simulink model "einMassenSchwingerAngeregt"  (R2017b)
settings: Solver=ode8  StartTime=0.0  StopTime=t_max  FixedStep=stepSize  RelTol=relTol
values from neighbouring files (symbols this model uses):
  c = 10    [Aufgabe2_parameterInit.m]
  d = .5    (= 0.5)    [Aufgabe2_parameterInit.m]
  m = 1    [Aufgabe2_parameterInit.m]
  y0 = 0    [Aufgabe2_parameterInit.m]
  yDot0 = 0    [Aufgabe2_parameterInit.m]
undefined symbols (not defined in the file or in its folder): F_sigma, omega, switchVar
settings Model: Creator=jens  LastModifiedBy=jens

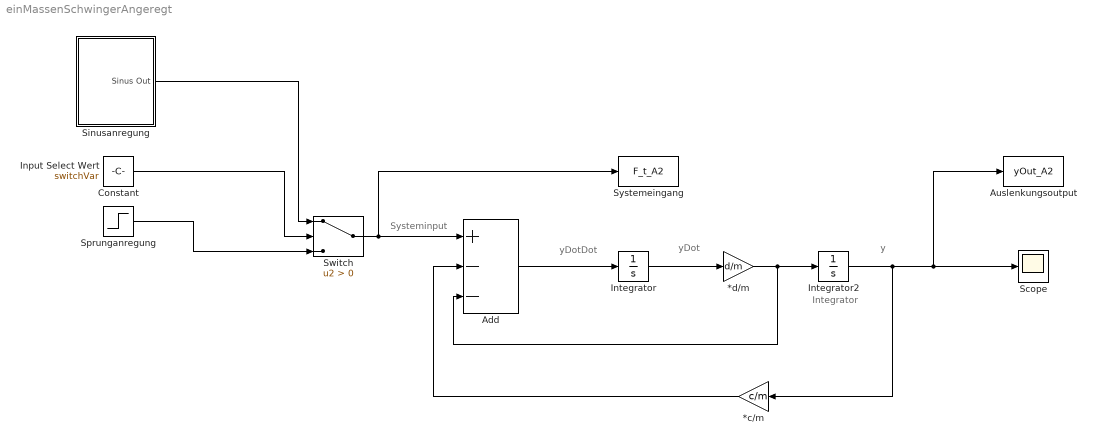
== system einMassenSchwingerAngeregt ==
  note: Integrator
  note: Systeminput
  note: yDotDot
  note: y
  note: yDot
  *c/m : Gain  Gain=c/m
  *d/m : Gain  Gain=d/m
  Add : Sum  Inputs=+--
  Auslenkungsoutput : ToWorkspace  VariableName=yOut_A2  SaveFormat=Timeseries  SampleTime=-1
  Constant : Constant
  Input Select Wert : Constant  Value=switchVar
  "Integrator " : Integrator  InitialCondition=yDot0
  Integrator2 : Integrator  InitialCondition=y0
  Scope : Scope
  Sinusanregung : Subsystem
  Sprunganregung : Step  After=F_sigma  SampleTime=0
  Switch : Switch  Criteria=u2 > Threshold
  Systemeingang : ToWorkspace  VariableName=F_t_A2  SaveFormat=Timeseries  SampleTime=-1
  wires:
  *d/m/1 -> Add/3, Integrator2/1
  Add/1 -> "Integrator "/1
  Integrator2/1 -> *c/m/1, Auslenkungsoutput/1, Scope/1
  "Integrator "/1 -> *d/m/1
  *c/m/1 -> Add/2
  Switch/1 -> Systemeingang/1, Add/1
  Sinusanregung/1(Sinus Out) -> Switch/1
  Sprunganregung/1 -> Switch/3
  Input Select Wert/1 -> Switch/2

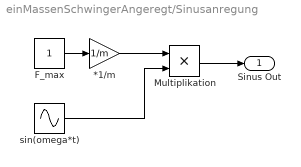
== system einMassenSchwingerAngeregt/Sinusanregung ==
  *1/m : Gain  Gain=1/m
  F_max : Constant
  Multiplikation : Product
  sin(omega*t) : Sin  Frequency=omega  SampleTime=0
  Sinus Out : Outport
  wires:
  sin(omega*t)/1 -> Multiplikation/2
  *1/m/1 -> Multiplikation/1
  Multiplikation/1 -> Sinus Out/1
  F_max/1 -> *1/m/1
